simulink model "mpm_blocks"  (R2023a)
settings: Solver=VariableStepAuto  StartTime=0.0  StopTime=10.0  RelTol=1e-3
undefined symbols (not defined in the file or in its folder): conv, es
(part 2 of 3)

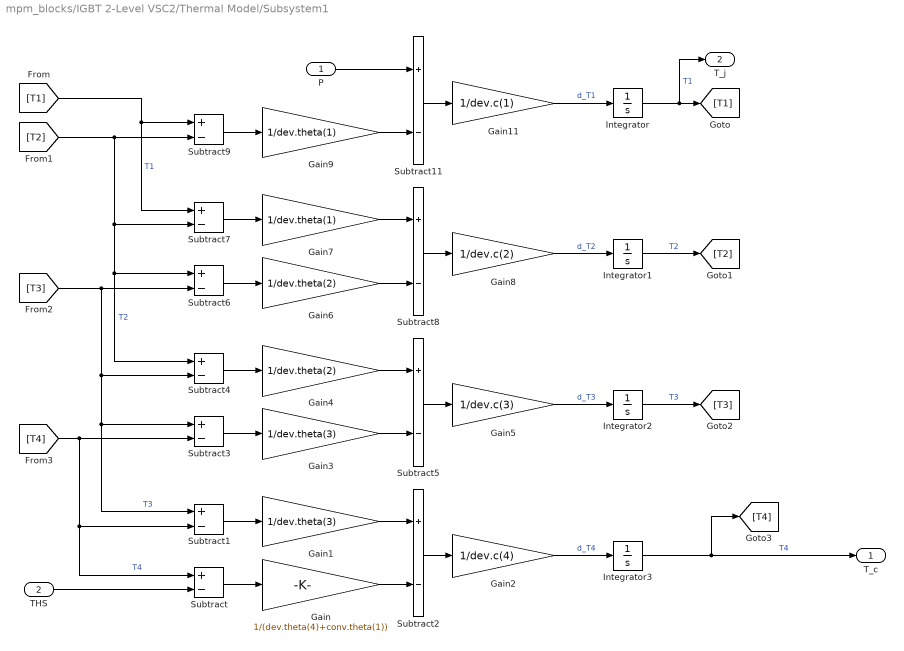
== system mpm_blocks/IGBT 2-Level VSC2/Thermal Model/Subsystem1 ==
  P : Inport
  THS : Inport  Port=2
  Gain : Gain  Gain=1/(dev.theta(4)+conv.theta(1))
  Gain1 : Gain  Gain=1/dev.theta(3)
  Gain11 : Gain  Gain=1/dev.c(1)
  Gain2 : Gain  Gain=1/dev.c(4)
  Gain3 : Gain  Gain=1/dev.theta(3)
  Gain4 : Gain  Gain=1/dev.theta(2)
  Gain5 : Gain  Gain=1/dev.c(3)
  Gain6 : Gain  Gain=1/dev.theta(2)
  Gain7 : Gain  Gain=1/dev.theta(1)
  Gain8 : Gain  Gain=1/dev.c(2)
  Gain9 : Gain  Gain=1/dev.theta(1)
  Integrator{,1..3} (4 alike) : Integrator  InitialCondition=conv.T_init-273.15
  Subtract{,1..9,11} (11 alike) : Sum  Inputs=+-
  T_c : Outport
  T_j : Outport  Port=2
  wires:
  Gain6/1 -> Subtract8/2
  Gain7/1 -> Subtract8/1
  Subtract11/1 -> Gain11/1
  Subtract6/1 -> Gain6/1
  Subtract2/1 -> Gain2/1
  Gain11/1 -> Integrator/1  "d_T1"
  Gain5/1 -> Integrator2/1  "d_T3"
  Integrator2/1 -> [T3]  "T3"
  Gain3/1 -> Subtract5/2
  Gain9/1 -> Subtract11/2
  Gain1/1 -> Subtract2/1
  THS/1 -> Subtract/2
  Subtract8/1 -> Gain8/1
  Gain2/1 -> Integrator3/1  "d_T4"
  Integrator3/1 -> T_c/1, [T4]  "T4"
  Subtract4/1 -> Gain4/1
  Subtract7/1 -> Gain7/1
  [T4] -> Subtract3/2, Subtract1/2, Subtract/1  "T4"
  Subtract/1 -> Gain/1
  Integrator1/1 -> [T2]  "T2"
  [T1] -> Subtract7/1, Subtract9/1  "T1"
  Subtract1/1 -> Gain1/1
  Subtract9/1 -> Gain9/1
  P/1 -> Subtract11/1
  [T3] -> Subtract6/2, Subtract4/2, Subtract3/1, Subtract1/1  "T3"
  Integrator/1 -> [T1], T_j/1  "T1"
  Gain8/1 -> Integrator1/1  "d_T2"
  Subtract3/1 -> Gain3/1
  Gain4/1 -> Subtract5/1
  Subtract5/1 -> Gain5/1
  Gain/1 -> Subtract2/2
  [T2] -> Subtract9/2, Subtract7/2, Subtract6/1, Subtract4/1  "T2"

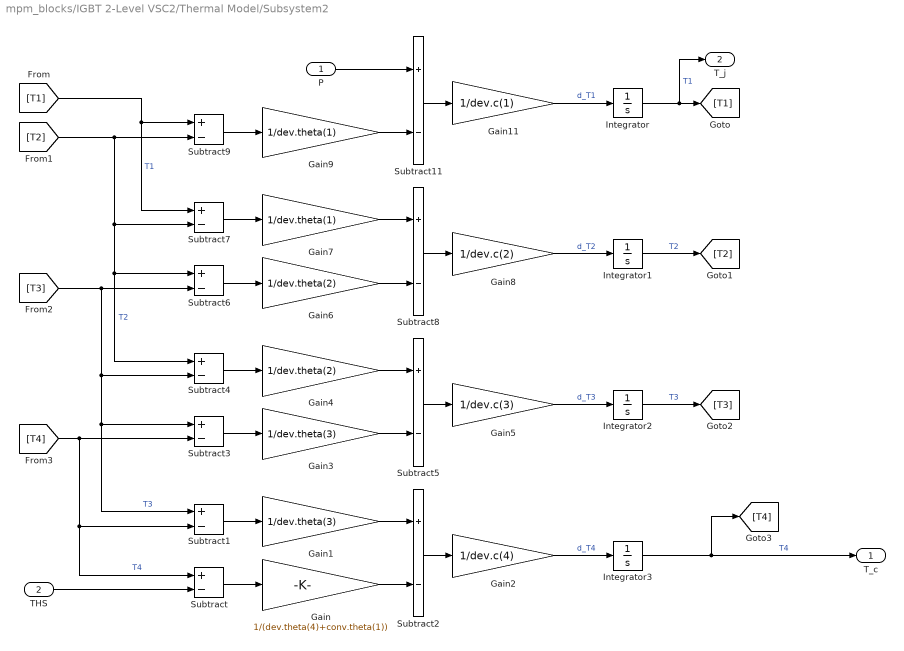
== system mpm_blocks/IGBT 2-Level VSC2/Thermal Model/Subsystem2 ==
  P : Inport
  THS : Inport  Port=2
  Gain : Gain  Gain=1/(dev.theta(4)+conv.theta(1))
  Gain1 : Gain  Gain=1/dev.theta(3)
  Gain11 : Gain  Gain=1/dev.c(1)
  Gain2 : Gain  Gain=1/dev.c(4)
  Gain3 : Gain  Gain=1/dev.theta(3)
  Gain4 : Gain  Gain=1/dev.theta(2)
  Gain5 : Gain  Gain=1/dev.c(3)
  Gain6 : Gain  Gain=1/dev.theta(2)
  Gain7 : Gain  Gain=1/dev.theta(1)
  Gain8 : Gain  Gain=1/dev.c(2)
  Gain9 : Gain  Gain=1/dev.theta(1)
  Integrator{,1..3} (4 alike) : Integrator  InitialCondition=conv.T_init-273.15
  Subtract{,1..9,11} (11 alike) : Sum  Inputs=+-
  T_c : Outport
  T_j : Outport  Port=2
  wires:
  Gain6/1 -> Subtract8/2
  Gain7/1 -> Subtract8/1
  Subtract11/1 -> Gain11/1
  Subtract6/1 -> Gain6/1
  Subtract2/1 -> Gain2/1
  Gain11/1 -> Integrator/1  "d_T1"
  Gain5/1 -> Integrator2/1  "d_T3"
  Integrator2/1 -> [T3]  "T3"
  Gain3/1 -> Subtract5/2
  Gain9/1 -> Subtract11/2
  Gain1/1 -> Subtract2/1
  THS/1 -> Subtract/2
  Subtract8/1 -> Gain8/1
  Gain2/1 -> Integrator3/1  "d_T4"
  Integrator3/1 -> T_c/1, [T4]  "T4"
  Subtract4/1 -> Gain4/1
  Subtract7/1 -> Gain7/1
  [T4] -> Subtract3/2, Subtract1/2, Subtract/1  "T4"
  Subtract/1 -> Gain/1
  Integrator1/1 -> [T2]  "T2"
  [T1] -> Subtract7/1, Subtract9/1  "T1"
  Subtract1/1 -> Gain1/1
  Subtract9/1 -> Gain9/1
  P/1 -> Subtract11/1
  [T3] -> Subtract6/2, Subtract4/2, Subtract3/1, Subtract1/1  "T3"
  Integrator/1 -> [T1], T_j/1  "T1"
  Gain8/1 -> Integrator1/1  "d_T2"
  Subtract3/1 -> Gain3/1
  Gain4/1 -> Subtract5/1
  Subtract5/1 -> Gain5/1
  Gain/1 -> Subtract2/2
  [T2] -> Subtract9/2, Subtract7/2, Subtract6/1, Subtract4/1  "T2"

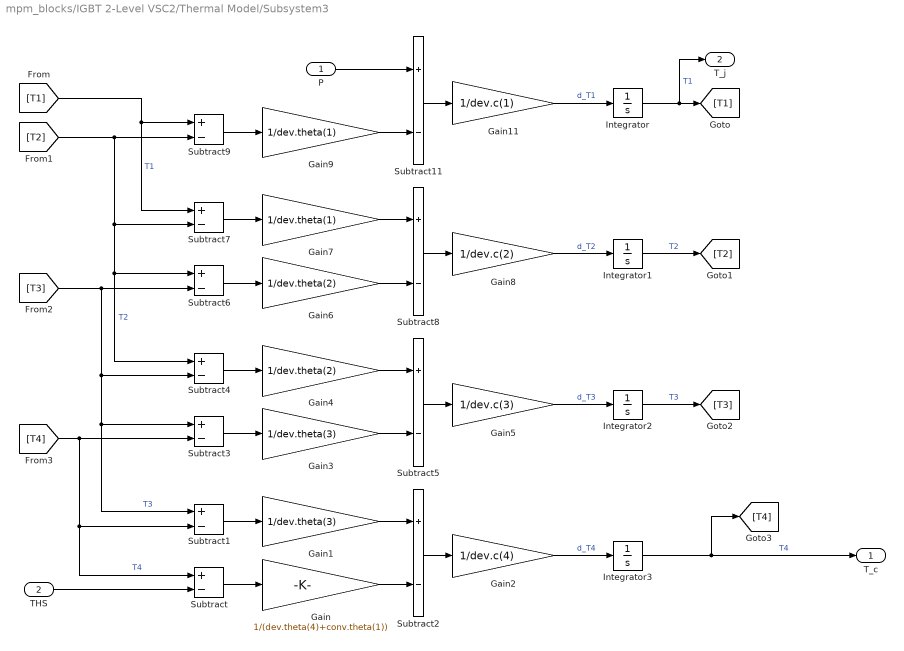
== system mpm_blocks/IGBT 2-Level VSC2/Thermal Model/Subsystem3 ==
  P : Inport
  THS : Inport  Port=2
  Gain : Gain  Gain=1/(dev.theta(4)+conv.theta(1))
  Gain1 : Gain  Gain=1/dev.theta(3)
  Gain11 : Gain  Gain=1/dev.c(1)
  Gain2 : Gain  Gain=1/dev.c(4)
  Gain3 : Gain  Gain=1/dev.theta(3)
  Gain4 : Gain  Gain=1/dev.theta(2)
  Gain5 : Gain  Gain=1/dev.c(3)
  Gain6 : Gain  Gain=1/dev.theta(2)
  Gain7 : Gain  Gain=1/dev.theta(1)
  Gain8 : Gain  Gain=1/dev.c(2)
  Gain9 : Gain  Gain=1/dev.theta(1)
  Integrator{,1..3} (4 alike) : Integrator  InitialCondition=conv.T_init-273.15
  Subtract{,1..9,11} (11 alike) : Sum  Inputs=+-
  T_c : Outport
  T_j : Outport  Port=2
  wires:
  Gain6/1 -> Subtract8/2
  Gain7/1 -> Subtract8/1
  Subtract11/1 -> Gain11/1
  Subtract6/1 -> Gain6/1
  Subtract2/1 -> Gain2/1
  Gain11/1 -> Integrator/1  "d_T1"
  Gain5/1 -> Integrator2/1  "d_T3"
  Integrator2/1 -> [T3]  "T3"
  Gain3/1 -> Subtract5/2
  Gain9/1 -> Subtract11/2
  Gain1/1 -> Subtract2/1
  THS/1 -> Subtract/2
  Subtract8/1 -> Gain8/1
  Gain2/1 -> Integrator3/1  "d_T4"
  Integrator3/1 -> T_c/1, [T4]  "T4"
  Subtract4/1 -> Gain4/1
  Subtract7/1 -> Gain7/1
  [T4] -> Subtract3/2, Subtract1/2, Subtract/1  "T4"
  Subtract/1 -> Gain/1
  Integrator1/1 -> [T2]  "T2"
  [T1] -> Subtract7/1, Subtract9/1  "T1"
  Subtract1/1 -> Gain1/1
  Subtract9/1 -> Gain9/1
  P/1 -> Subtract11/1
  [T3] -> Subtract6/2, Subtract4/2, Subtract3/1, Subtract1/1  "T3"
  Integrator/1 -> [T1], T_j/1  "T1"
  Gain8/1 -> Integrator1/1  "d_T2"
  Subtract3/1 -> Gain3/1
  Gain4/1 -> Subtract5/1
  Subtract5/1 -> Gain5/1
  Gain/1 -> Subtract2/2
  [T2] -> Subtract9/2, Subtract7/2, Subtract6/1, Subtract4/1  "T2"

== system mpm_blocks/IGBT 2-Level VSC2/Thermal Model/Subsystem4 ==
  P : Inport
  THS : Inport  Port=2
  Gain : Gain  Gain=1/(dev.theta(4)+conv.theta(1))
  Gain1 : Gain  Gain=1/dev.theta(3)
  Gain11 : Gain  Gain=1/dev.c(1)
  Gain2 : Gain  Gain=1/dev.c(4)
  Gain3 : Gain  Gain=1/dev.theta(3)
  Gain4 : Gain  Gain=1/dev.theta(2)
  Gain5 : Gain  Gain=1/dev.c(3)
  Gain6 : Gain  Gain=1/dev.theta(2)
  Gain7 : Gain  Gain=1/dev.theta(1)
  Gain8 : Gain  Gain=1/dev.c(2)
  Gain9 : Gain  Gain=1/dev.theta(1)
  Integrator{,1..3} (4 alike) : Integrator  InitialCondition=conv.T_init-273.15
  Subtract{,1..9,11} (11 alike) : Sum  Inputs=+-
  T_c : Outport
  T_j : Outport  Port=2
  wires:
  Gain6/1 -> Subtract8/2
  Gain7/1 -> Subtract8/1
  Subtract11/1 -> Gain11/1
  Subtract6/1 -> Gain6/1
  Subtract2/1 -> Gain2/1
  Gain11/1 -> Integrator/1  "d_T1"
  Gain5/1 -> Integrator2/1  "d_T3"
  Integrator2/1 -> [T3]  "T3"
  Gain3/1 -> Subtract5/2
  Gain9/1 -> Subtract11/2
  Gain1/1 -> Subtract2/1
  THS/1 -> Subtract/2
  Subtract8/1 -> Gain8/1
  Gain2/1 -> Integrator3/1  "d_T4"
  Integrator3/1 -> T_c/1, [T4]  "T4"
  Subtract4/1 -> Gain4/1
  Subtract7/1 -> Gain7/1
  [T4] -> Subtract3/2, Subtract1/2, Subtract/1  "T4"
  Subtract/1 -> Gain/1
  Integrator1/1 -> [T2]  "T2"
  [T1] -> Subtract7/1, Subtract9/1  "T1"
  Subtract1/1 -> Gain1/1
  Subtract9/1 -> Gain9/1
  P/1 -> Subtract11/1
  [T3] -> Subtract6/2, Subtract4/2, Subtract3/1, Subtract1/1  "T3"
  Integrator/1 -> [T1], T_j/1  "T1"
  Gain8/1 -> Integrator1/1  "d_T2"
  Subtract3/1 -> Gain3/1
  Gain4/1 -> Subtract5/1
  Subtract5/1 -> Gain5/1
  Gain/1 -> Subtract2/2
  [T2] -> Subtract9/2, Subtract7/2, Subtract6/1, Subtract4/1  "T2"

== system mpm_blocks/IGBT 2-Level VSC2/Thermal Model/Subsystem5 ==
  P : Inport
  THS : Inport  Port=2
  Gain : Gain  Gain=1/(dev.theta(4)+conv.theta(1))
  Gain1 : Gain  Gain=1/dev.theta(3)
  Gain11 : Gain  Gain=1/dev.c(1)
  Gain2 : Gain  Gain=1/dev.c(4)
  Gain3 : Gain  Gain=1/dev.theta(3)
  Gain4 : Gain  Gain=1/dev.theta(2)
  Gain5 : Gain  Gain=1/dev.c(3)
  Gain6 : Gain  Gain=1/dev.theta(2)
  Gain7 : Gain  Gain=1/dev.theta(1)
  Gain8 : Gain  Gain=1/dev.c(2)
  Gain9 : Gain  Gain=1/dev.theta(1)
  Integrator{,1..3} (4 alike) : Integrator  InitialCondition=conv.T_init-273.15
  Subtract{,1..9,11} (11 alike) : Sum  Inputs=+-
  T_c : Outport
  T_j : Outport  Port=2
  wires:
  Gain6/1 -> Subtract8/2
  Gain7/1 -> Subtract8/1
  Subtract11/1 -> Gain11/1
  Subtract6/1 -> Gain6/1
  Subtract2/1 -> Gain2/1
  Gain11/1 -> Integrator/1  "d_T1"
  Gain5/1 -> Integrator2/1  "d_T3"
  Integrator2/1 -> [T3]  "T3"
  Gain3/1 -> Subtract5/2
  Gain9/1 -> Subtract11/2
  Gain1/1 -> Subtract2/1
  THS/1 -> Subtract/2
  Subtract8/1 -> Gain8/1
  Gain2/1 -> Integrator3/1  "d_T4"
  Integrator3/1 -> T_c/1, [T4]  "T4"
  Subtract4/1 -> Gain4/1
  Subtract7/1 -> Gain7/1
  [T4] -> Subtract3/2, Subtract1/2, Subtract/1  "T4"
  Subtract/1 -> Gain/1
  Integrator1/1 -> [T2]  "T2"
  [T1] -> Subtract7/1, Subtract9/1  "T1"
  Subtract1/1 -> Gain1/1
  Subtract9/1 -> Gain9/1
  P/1 -> Subtract11/1
  [T3] -> Subtract6/2, Subtract4/2, Subtract3/1, Subtract1/1  "T3"
  Integrator/1 -> [T1], T_j/1  "T1"
  Gain8/1 -> Integrator1/1  "d_T2"
  Subtract3/1 -> Gain3/1
  Gain4/1 -> Subtract5/1
  Subtract5/1 -> Gain5/1
  Gain/1 -> Subtract2/2
  [T2] -> Subtract9/2, Subtract7/2, Subtract6/1, Subtract4/1  "T2"

== system mpm_blocks/IGBT 2-Level VSC2/Thermal Model/Subsystem6 ==
  P : Inport
  THS : Inport  Port=2
  Gain : Gain  Gain=1/(dev.theta(4)+conv.theta(1))
  Gain1 : Gain  Gain=1/dev.theta(3)
  Gain11 : Gain  Gain=1/dev.c(1)
  Gain2 : Gain  Gain=1/dev.c(4)
  Gain3 : Gain  Gain=1/dev.theta(3)
  Gain4 : Gain  Gain=1/dev.theta(2)
  Gain5 : Gain  Gain=1/dev.c(3)
  Gain6 : Gain  Gain=1/dev.theta(2)
  Gain7 : Gain  Gain=1/dev.theta(1)
  Gain8 : Gain  Gain=1/dev.c(2)
  Gain9 : Gain  Gain=1/dev.theta(1)
  Integrator{,1..3} (4 alike) : Integrator  InitialCondition=conv.T_init-273.15
  Subtract{,1..9,11} (11 alike) : Sum  Inputs=+-
  T_c : Outport
  T_j : Outport  Port=2
  wires:
  Gain6/1 -> Subtract8/2
  Gain7/1 -> Subtract8/1
  Subtract11/1 -> Gain11/1
  Subtract6/1 -> Gain6/1
  Subtract2/1 -> Gain2/1
  Gain11/1 -> Integrator/1  "d_T1"
  Gain5/1 -> Integrator2/1  "d_T3"
  Integrator2/1 -> [T3]  "T3"
  Gain3/1 -> Subtract5/2
  Gain9/1 -> Subtract11/2
  Gain1/1 -> Subtract2/1
  THS/1 -> Subtract/2
  Subtract8/1 -> Gain8/1
  Gain2/1 -> Integrator3/1  "d_T4"
  Integrator3/1 -> T_c/1, [T4]  "T4"
  Subtract4/1 -> Gain4/1
  Subtract7/1 -> Gain7/1
  [T4] -> Subtract3/2, Subtract1/2, Subtract/1  "T4"
  Subtract/1 -> Gain/1
  Integrator1/1 -> [T2]  "T2"
  [T1] -> Subtract7/1, Subtract9/1  "T1"
  Subtract1/1 -> Gain1/1
  Subtract9/1 -> Gain9/1
  P/1 -> Subtract11/1
  [T3] -> Subtract6/2, Subtract4/2, Subtract3/1, Subtract1/1  "T3"
  Integrator/1 -> [T1], T_j/1  "T1"
  Gain8/1 -> Integrator1/1  "d_T2"
  Subtract3/1 -> Gain3/1
  Gain4/1 -> Subtract5/1
  Subtract5/1 -> Gain5/1
  Gain/1 -> Subtract2/2
  [T2] -> Subtract9/2, Subtract7/2, Subtract6/1, Subtract4/1  "T2"

== system mpm_blocks/IGBT 2-Level VSC2/Thermal Model1/Subsystem1 ==
  P : Inport
  THS : Inport  Port=2
  Gain : Gain  Gain=1/(dev.theta(4)+conv.theta(1))
  Gain1 : Gain  Gain=1/dev.theta(3)
  Gain11 : Gain  Gain=1/dev.c(1)
  Gain2 : Gain  Gain=1/dev.c(4)
  Gain3 : Gain  Gain=1/dev.theta(3)
  Gain4 : Gain  Gain=1/dev.theta(2)
  Gain5 : Gain  Gain=1/dev.c(3)
  Gain6 : Gain  Gain=1/dev.theta(2)
  Gain7 : Gain  Gain=1/dev.theta(1)
  Gain8 : Gain  Gain=1/dev.c(2)
  Gain9 : Gain  Gain=1/dev.theta(1)
  Integrator{,1..3} (4 alike) : Integrator  InitialCondition=conv.T_init-273.15
  Subtract{,1..9,11} (11 alike) : Sum  Inputs=+-
  T_c : Outport
  T_j : Outport  Port=2
  wires:
  [T2] -> Subtract4/1, Subtract6/1, Subtract7/2, Subtract9/2  "T2"
  Gain/1 -> Subtract2/2
  Subtract5/1 -> Gain5/1
  Gain4/1 -> Subtract5/1
  Subtract3/1 -> Gain3/1
  Gain8/1 -> Integrator1/1  "d_T2"
  Integrator/1 -> T_j/1, [T1]  "T1"
  [T3] -> Subtract1/1, Subtract3/1, Subtract4/2, Subtract6/2  "T3"
  P/1 -> Subtract11/1
  Subtract9/1 -> Gain9/1
  Subtract1/1 -> Gain1/1
  [T1] -> Subtract9/1, Subtract7/1  "T1"
  Integrator1/1 -> [T2]  "T2"
  Subtract/1 -> Gain/1
  [T4] -> Subtract/1, Subtract1/2, Subtract3/2  "T4"
  Subtract7/1 -> Gain7/1
  Subtract4/1 -> Gain4/1
  Integrator3/1 -> [T4], T_c/1  "T4"
  Gain2/1 -> Integrator3/1  "d_T4"
  Subtract8/1 -> Gain8/1
  THS/1 -> Subtract/2
  Gain1/1 -> Subtract2/1
  Gain9/1 -> Subtract11/2
  Gain3/1 -> Subtract5/2
  Integrator2/1 -> [T3]  "T3"
  Gain5/1 -> Integrator2/1  "d_T3"
  Gain11/1 -> Integrator/1  "d_T1"
  Subtract2/1 -> Gain2/1
  Subtract6/1 -> Gain6/1
  Subtract11/1 -> Gain11/1
  Gain7/1 -> Subtract8/1
  Gain6/1 -> Subtract8/2

== system mpm_blocks/IGBT 2-Level VSC2/Thermal Model1/Subsystem2 ==
  P : Inport
  THS : Inport  Port=2
  Gain : Gain  Gain=1/(dev.theta(4)+conv.theta(1))
  Gain1 : Gain  Gain=1/dev.theta(3)
  Gain11 : Gain  Gain=1/dev.c(1)
  Gain2 : Gain  Gain=1/dev.c(4)
  Gain3 : Gain  Gain=1/dev.theta(3)
  Gain4 : Gain  Gain=1/dev.theta(2)
  Gain5 : Gain  Gain=1/dev.c(3)
  Gain6 : Gain  Gain=1/dev.theta(2)
  Gain7 : Gain  Gain=1/dev.theta(1)
  Gain8 : Gain  Gain=1/dev.c(2)
  Gain9 : Gain  Gain=1/dev.theta(1)
  Integrator{,1..3} (4 alike) : Integrator  InitialCondition=conv.T_init-273.15
  Subtract{,1..9,11} (11 alike) : Sum  Inputs=+-
  T_c : Outport
  T_j : Outport  Port=2
  wires:
  [T2] -> Subtract4/1, Subtract6/1, Subtract7/2, Subtract9/2  "T2"
  Gain/1 -> Subtract2/2
  Subtract5/1 -> Gain5/1
  Gain4/1 -> Subtract5/1
  Subtract3/1 -> Gain3/1
  Gain8/1 -> Integrator1/1  "d_T2"
  Integrator/1 -> T_j/1, [T1]  "T1"
  [T3] -> Subtract1/1, Subtract3/1, Subtract4/2, Subtract6/2  "T3"
  P/1 -> Subtract11/1
  Subtract9/1 -> Gain9/1
  Subtract1/1 -> Gain1/1
  [T1] -> Subtract9/1, Subtract7/1  "T1"
  Integrator1/1 -> [T2]  "T2"
  Subtract/1 -> Gain/1
  [T4] -> Subtract/1, Subtract1/2, Subtract3/2  "T4"
  Subtract7/1 -> Gain7/1
  Subtract4/1 -> Gain4/1
  Integrator3/1 -> [T4], T_c/1  "T4"
  Gain2/1 -> Integrator3/1  "d_T4"
  Subtract8/1 -> Gain8/1
  THS/1 -> Subtract/2
  Gain1/1 -> Subtract2/1
  Gain9/1 -> Subtract11/2
  Gain3/1 -> Subtract5/2
  Integrator2/1 -> [T3]  "T3"
  Gain5/1 -> Integrator2/1  "d_T3"
  Gain11/1 -> Integrator/1  "d_T1"
  Subtract2/1 -> Gain2/1
  Subtract6/1 -> Gain6/1
  Subtract11/1 -> Gain11/1
  Gain7/1 -> Subtract8/1
  Gain6/1 -> Subtract8/2

== system mpm_blocks/IGBT 2-Level VSC2/Thermal Model1/Subsystem3 ==
  P : Inport
  THS : Inport  Port=2
  Gain : Gain  Gain=1/(dev.theta(4)+conv.theta(1))
  Gain1 : Gain  Gain=1/dev.theta(3)
  Gain11 : Gain  Gain=1/dev.c(1)
  Gain2 : Gain  Gain=1/dev.c(4)
  Gain3 : Gain  Gain=1/dev.theta(3)
  Gain4 : Gain  Gain=1/dev.theta(2)
  Gain5 : Gain  Gain=1/dev.c(3)
  Gain6 : Gain  Gain=1/dev.theta(2)
  Gain7 : Gain  Gain=1/dev.theta(1)
  Gain8 : Gain  Gain=1/dev.c(2)
  Gain9 : Gain  Gain=1/dev.theta(1)
  Integrator{,1..3} (4 alike) : Integrator  InitialCondition=conv.T_init-273.15
  Subtract{,1..9,11} (11 alike) : Sum  Inputs=+-
  T_c : Outport
  T_j : Outport  Port=2
  wires:
  [T2] -> Subtract4/1, Subtract6/1, Subtract7/2, Subtract9/2  "T2"
  Gain/1 -> Subtract2/2
  Subtract5/1 -> Gain5/1
  Gain4/1 -> Subtract5/1
  Subtract3/1 -> Gain3/1
  Gain8/1 -> Integrator1/1  "d_T2"
  Integrator/1 -> T_j/1, [T1]  "T1"
  [T3] -> Subtract1/1, Subtract3/1, Subtract4/2, Subtract6/2  "T3"
  P/1 -> Subtract11/1
  Subtract9/1 -> Gain9/1
  Subtract1/1 -> Gain1/1
  [T1] -> Subtract9/1, Subtract7/1  "T1"
  Integrator1/1 -> [T2]  "T2"
  Subtract/1 -> Gain/1
  [T4] -> Subtract/1, Subtract1/2, Subtract3/2  "T4"
  Subtract7/1 -> Gain7/1
  Subtract4/1 -> Gain4/1
  Integrator3/1 -> [T4], T_c/1  "T4"
  Gain2/1 -> Integrator3/1  "d_T4"
  Subtract8/1 -> Gain8/1
  THS/1 -> Subtract/2
  Gain1/1 -> Subtract2/1
  Gain9/1 -> Subtract11/2
  Gain3/1 -> Subtract5/2
  Integrator2/1 -> [T3]  "T3"
  Gain5/1 -> Integrator2/1  "d_T3"
  Gain11/1 -> Integrator/1  "d_T1"
  Subtract2/1 -> Gain2/1
  Subtract6/1 -> Gain6/1
  Subtract11/1 -> Gain11/1
  Gain7/1 -> Subtract8/1
  Gain6/1 -> Subtract8/2

== system mpm_blocks/IGBT 2-Level VSC2/Thermal Model1/Subsystem4 ==
  P : Inport
  THS : Inport  Port=2
  Gain : Gain  Gain=1/(dev.theta(4)+conv.theta(1))
  Gain1 : Gain  Gain=1/dev.theta(3)
  Gain11 : Gain  Gain=1/dev.c(1)
  Gain2 : Gain  Gain=1/dev.c(4)
  Gain3 : Gain  Gain=1/dev.theta(3)
  Gain4 : Gain  Gain=1/dev.theta(2)
  Gain5 : Gain  Gain=1/dev.c(3)
  Gain6 : Gain  Gain=1/dev.theta(2)
  Gain7 : Gain  Gain=1/dev.theta(1)
  Gain8 : Gain  Gain=1/dev.c(2)
  Gain9 : Gain  Gain=1/dev.theta(1)
  Integrator{,1..3} (4 alike) : Integrator  InitialCondition=conv.T_init-273.15
  Subtract{,1..9,11} (11 alike) : Sum  Inputs=+-
  T_c : Outport
  T_j : Outport  Port=2
  wires:
  [T2] -> Subtract4/1, Subtract6/1, Subtract7/2, Subtract9/2  "T2"
  Gain/1 -> Subtract2/2
  Subtract5/1 -> Gain5/1
  Gain4/1 -> Subtract5/1
  Subtract3/1 -> Gain3/1
  Gain8/1 -> Integrator1/1  "d_T2"
  Integrator/1 -> T_j/1, [T1]  "T1"
  [T3] -> Subtract1/1, Subtract3/1, Subtract4/2, Subtract6/2  "T3"
  P/1 -> Subtract11/1
  Subtract9/1 -> Gain9/1
  Subtract1/1 -> Gain1/1
  [T1] -> Subtract9/1, Subtract7/1  "T1"
  Integrator1/1 -> [T2]  "T2"
  Subtract/1 -> Gain/1
  [T4] -> Subtract/1, Subtract1/2, Subtract3/2  "T4"
  Subtract7/1 -> Gain7/1
  Subtract4/1 -> Gain4/1
  Integrator3/1 -> [T4], T_c/1  "T4"
  Gain2/1 -> Integrator3/1  "d_T4"
  Subtract8/1 -> Gain8/1
  THS/1 -> Subtract/2
  Gain1/1 -> Subtract2/1
  Gain9/1 -> Subtract11/2
  Gain3/1 -> Subtract5/2
  Integrator2/1 -> [T3]  "T3"
  Gain5/1 -> Integrator2/1  "d_T3"
  Gain11/1 -> Integrator/1  "d_T1"
  Subtract2/1 -> Gain2/1
  Subtract6/1 -> Gain6/1
  Subtract11/1 -> Gain11/1
  Gain7/1 -> Subtract8/1
  Gain6/1 -> Subtract8/2

== system mpm_blocks/IGBT 2-Level VSC2/Thermal Model1/Subsystem5 ==
  P : Inport
  THS : Inport  Port=2
  Gain : Gain  Gain=1/(dev.theta(4)+conv.theta(1))
  Gain1 : Gain  Gain=1/dev.theta(3)
  Gain11 : Gain  Gain=1/dev.c(1)
  Gain2 : Gain  Gain=1/dev.c(4)
  Gain3 : Gain  Gain=1/dev.theta(3)
  Gain4 : Gain  Gain=1/dev.theta(2)
  Gain5 : Gain  Gain=1/dev.c(3)
  Gain6 : Gain  Gain=1/dev.theta(2)
  Gain7 : Gain  Gain=1/dev.theta(1)
  Gain8 : Gain  Gain=1/dev.c(2)
  Gain9 : Gain  Gain=1/dev.theta(1)
  Integrator{,1..3} (4 alike) : Integrator  InitialCondition=conv.T_init-273.15
  Subtract{,1..9,11} (11 alike) : Sum  Inputs=+-
  T_c : Outport
  T_j : Outport  Port=2
  wires:
  [T2] -> Subtract4/1, Subtract6/1, Subtract7/2, Subtract9/2  "T2"
  Gain/1 -> Subtract2/2
  Subtract5/1 -> Gain5/1
  Gain4/1 -> Subtract5/1
  Subtract3/1 -> Gain3/1
  Gain8/1 -> Integrator1/1  "d_T2"
  Integrator/1 -> T_j/1, [T1]  "T1"
  [T3] -> Subtract1/1, Subtract3/1, Subtract4/2, Subtract6/2  "T3"
  P/1 -> Subtract11/1
  Subtract9/1 -> Gain9/1
  Subtract1/1 -> Gain1/1
  [T1] -> Subtract9/1, Subtract7/1  "T1"
  Integrator1/1 -> [T2]  "T2"
  Subtract/1 -> Gain/1
  [T4] -> Subtract/1, Subtract1/2, Subtract3/2  "T4"
  Subtract7/1 -> Gain7/1
  Subtract4/1 -> Gain4/1
  Integrator3/1 -> [T4], T_c/1  "T4"
  Gain2/1 -> Integrator3/1  "d_T4"
  Subtract8/1 -> Gain8/1
  THS/1 -> Subtract/2
  Gain1/1 -> Subtract2/1
  Gain9/1 -> Subtract11/2
  Gain3/1 -> Subtract5/2
  Integrator2/1 -> [T3]  "T3"
  Gain5/1 -> Integrator2/1  "d_T3"
  Gain11/1 -> Integrator/1  "d_T1"
  Subtract2/1 -> Gain2/1
  Subtract6/1 -> Gain6/1
  Subtract11/1 -> Gain11/1
  Gain7/1 -> Subtract8/1
  Gain6/1 -> Subtract8/2

== system mpm_blocks/IGBT 2-Level VSC2/Thermal Model1/Subsystem6 ==
  P : Inport
  THS : Inport  Port=2
  Gain : Gain  Gain=1/(dev.theta(4)+conv.theta(1))
  Gain1 : Gain  Gain=1/dev.theta(3)
  Gain11 : Gain  Gain=1/dev.c(1)
  Gain2 : Gain  Gain=1/dev.c(4)
  Gain3 : Gain  Gain=1/dev.theta(3)
  Gain4 : Gain  Gain=1/dev.theta(2)
  Gain5 : Gain  Gain=1/dev.c(3)
  Gain6 : Gain  Gain=1/dev.theta(2)
  Gain7 : Gain  Gain=1/dev.theta(1)
  Gain8 : Gain  Gain=1/dev.c(2)
  Gain9 : Gain  Gain=1/dev.theta(1)
  Integrator{,1..3} (4 alike) : Integrator  InitialCondition=conv.T_init-273.15
  Subtract{,1..9,11} (11 alike) : Sum  Inputs=+-
  T_c : Outport
  T_j : Outport  Port=2
  wires:
  [T2] -> Subtract4/1, Subtract6/1, Subtract7/2, Subtract9/2  "T2"
  Gain/1 -> Subtract2/2
  Subtract5/1 -> Gain5/1
  Gain4/1 -> Subtract5/1
  Subtract3/1 -> Gain3/1
  Gain8/1 -> Integrator1/1  "d_T2"
  Integrator/1 -> T_j/1, [T1]  "T1"
  [T3] -> Subtract1/1, Subtract3/1, Subtract4/2, Subtract6/2  "T3"
  P/1 -> Subtract11/1
  Subtract9/1 -> Gain9/1
  Subtract1/1 -> Gain1/1
  [T1] -> Subtract9/1, Subtract7/1  "T1"
  Integrator1/1 -> [T2]  "T2"
  Subtract/1 -> Gain/1
  [T4] -> Subtract/1, Subtract1/2, Subtract3/2  "T4"
  Subtract7/1 -> Gain7/1
  Subtract4/1 -> Gain4/1
  Integrator3/1 -> [T4], T_c/1  "T4"
  Gain2/1 -> Integrator3/1  "d_T4"
  Subtract8/1 -> Gain8/1
  THS/1 -> Subtract/2
  Gain1/1 -> Subtract2/1
  Gain9/1 -> Subtract11/2
  Gain3/1 -> Subtract5/2
  Integrator2/1 -> [T3]  "T3"
  Gain5/1 -> Integrator2/1  "d_T3"
  Gain11/1 -> Integrator/1  "d_T1"
  Subtract2/1 -> Gain2/1
  Subtract6/1 -> Gain6/1
  Subtract11/1 -> Gain11/1
  Gain7/1 -> Subtract8/1
  Gain6/1 -> Subtract8/2

== system mpm_blocks/MOSFET w// External Diode 2-Level VSC/Calculate Duty & Currents/Duty Cycle Estimation ==
  v_dc : Inport
  v_s : Inport  Port=2
  Constant : Constant
  Constant2 : Constant
  Constant3 : Constant  Value=2*conv.t_d*conv.f_sw
  Constant4 : Constant  Value=2*conv.t_d*conv.f_sw
  Divide : Product  Inputs=*/
  Gain : Gain  Gain=1/2
  Gain2 : Gain  Gain=2
  MATLAB Function : MATLAB Function  Commented=on  TreatAsAtomicUnit=on
  MATLAB Function3 : MATLAB Function  TreatAsAtomicUnit=on
  Mux : Mux  Inputs=[3 3]
  Mux1 : Mux  Inputs=3
  Selector : Selector  InputPortWidth=7  IndexOptions=Index vector (dialog)  Indices=[1 4 7]  OutputSizes=1
  Subtract : Sum  Inputs=-+-
  Sum of Elements : Sum  Inputs=+
  Sum1 : Sum  Inputs=+-+
  d_M : Outport
  d_deadTime : Outport  Port=2
  wires:
  MATLAB Function3/1(y) -> Sum1/3
  Constant/1 -> Sum1/1
  v_s/1 -> Gain2/1  "v_s"
  Constant2/1 -> Subtract/2
  Gain/1 -> Subtract/1, Mux/1, Mux1/1, MATLAB Function/1(d1)  "d_H"
  Divide/1 -> MATLAB Function3/1(u)  "m_a"
  Sum1/1 -> Gain/1
  Constant4/1 -> Mux1/3, MATLAB Function/3(d3), d_deadTime/1, Subtract/3  "d_deadTime"
  Subtract/1 -> Mux/2, Mux1/2, MATLAB Function/2(d2)  "d_L"
  Constant3/1 -> Sum1/2
  Mux/1 -> d_M/1
  Gain2/1 -> Divide/1
  v_dc/1 -> Divide/2
  Mux1/1 -> Selector/1
  Sum of Elements/1 -> ?  "dsum"
  Selector/1 -> Sum of Elements/1

== system mpm_blocks/MOSFET w// External Diode 2-Level VSC/Thermal Model/Subsystem1 ==
  P : Inport
  THS : Inport  Port=2
  Gain : Gain  Gain=1/(dev.theta(4)+conv.theta(1))
  Gain1 : Gain  Gain=1/dev.theta(3)
  Gain11 : Gain  Gain=1/dev.c(1)
  Gain2 : Gain  Gain=1/dev.c(4)
  Gain3 : Gain  Gain=1/dev.theta(3)
  Gain4 : Gain  Gain=1/dev.theta(2)
  Gain5 : Gain  Gain=1/dev.c(3)
  Gain6 : Gain  Gain=1/dev.theta(2)
  Gain7 : Gain  Gain=1/dev.theta(1)
  Gain8 : Gain  Gain=1/dev.c(2)
  Gain9 : Gain  Gain=1/dev.theta(1)
  Integrator{,1..3} (4 alike) : Integrator  InitialCondition=conv.T_init-273.15
  Subtract{,1..9,11} (11 alike) : Sum  Inputs=+-
  T_c : Outport
  T_j : Outport  Port=2
  wires:
  [T2] -> Subtract4/1, Subtract6/1, Subtract7/2, Subtract9/2  "T2"
  Gain/1 -> Subtract2/2
  Subtract5/1 -> Gain5/1
  Gain4/1 -> Subtract5/1
  Subtract3/1 -> Gain3/1
  Gain8/1 -> Integrator1/1  "d_T2"
  Integrator/1 -> T_j/1, [T1]  "T1"
  [T3] -> Subtract1/1, Subtract3/1, Subtract4/2, Subtract6/2  "T3"
  P/1 -> Subtract11/1
  Subtract9/1 -> Gain9/1
  Subtract1/1 -> Gain1/1
  [T1] -> Subtract9/1, Subtract7/1  "T1"
  Integrator1/1 -> [T2]  "T2"
  Subtract/1 -> Gain/1
  [T4] -> Subtract/1, Subtract1/2, Subtract3/2  "T4"
  Subtract7/1 -> Gain7/1
  Subtract4/1 -> Gain4/1
  Integrator3/1 -> [T4], T_c/1  "T4"
  Gain2/1 -> Integrator3/1  "d_T4"
  Subtract8/1 -> Gain8/1
  THS/1 -> Subtract/2
  Gain1/1 -> Subtract2/1
  Gain9/1 -> Subtract11/2
  Gain3/1 -> Subtract5/2
  Integrator2/1 -> [T3]  "T3"
  Gain5/1 -> Integrator2/1  "d_T3"
  Gain11/1 -> Integrator/1  "d_T1"
  Subtract2/1 -> Gain2/1
  Subtract6/1 -> Gain6/1
  Subtract11/1 -> Gain11/1
  Gain7/1 -> Subtract8/1
  Gain6/1 -> Subtract8/2

== system mpm_blocks/MOSFET w// External Diode 2-Level VSC/Thermal Model/Subsystem2 ==
  P : Inport
  THS : Inport  Port=2
  Gain : Gain  Gain=1/(dev.theta(4)+conv.theta(1))
  Gain1 : Gain  Gain=1/dev.theta(3)
  Gain11 : Gain  Gain=1/dev.c(1)
  Gain2 : Gain  Gain=1/dev.c(4)
  Gain3 : Gain  Gain=1/dev.theta(3)
  Gain4 : Gain  Gain=1/dev.theta(2)
  Gain5 : Gain  Gain=1/dev.c(3)
  Gain6 : Gain  Gain=1/dev.theta(2)
  Gain7 : Gain  Gain=1/dev.theta(1)
  Gain8 : Gain  Gain=1/dev.c(2)
  Gain9 : Gain  Gain=1/dev.theta(1)
  Integrator{,1..3} (4 alike) : Integrator  InitialCondition=conv.T_init-273.15
  Subtract{,1..9,11} (11 alike) : Sum  Inputs=+-
  T_c : Outport
  T_j : Outport  Port=2
  wires:
  [T2] -> Subtract4/1, Subtract6/1, Subtract7/2, Subtract9/2  "T2"
  Gain/1 -> Subtract2/2
  Subtract5/1 -> Gain5/1
  Gain4/1 -> Subtract5/1
  Subtract3/1 -> Gain3/1
  Gain8/1 -> Integrator1/1  "d_T2"
  Integrator/1 -> T_j/1, [T1]  "T1"
  [T3] -> Subtract1/1, Subtract3/1, Subtract4/2, Subtract6/2  "T3"
  P/1 -> Subtract11/1
  Subtract9/1 -> Gain9/1
  Subtract1/1 -> Gain1/1
  [T1] -> Subtract9/1, Subtract7/1  "T1"
  Integrator1/1 -> [T2]  "T2"
  Subtract/1 -> Gain/1
  [T4] -> Subtract/1, Subtract1/2, Subtract3/2  "T4"
  Subtract7/1 -> Gain7/1
  Subtract4/1 -> Gain4/1
  Integrator3/1 -> [T4], T_c/1  "T4"
  Gain2/1 -> Integrator3/1  "d_T4"
  Subtract8/1 -> Gain8/1
  THS/1 -> Subtract/2
  Gain1/1 -> Subtract2/1
  Gain9/1 -> Subtract11/2
  Gain3/1 -> Subtract5/2
  Integrator2/1 -> [T3]  "T3"
  Gain5/1 -> Integrator2/1  "d_T3"
  Gain11/1 -> Integrator/1  "d_T1"
  Subtract2/1 -> Gain2/1
  Subtract6/1 -> Gain6/1
  Subtract11/1 -> Gain11/1
  Gain7/1 -> Subtract8/1
  Gain6/1 -> Subtract8/2

== system mpm_blocks/MOSFET w// External Diode 2-Level VSC/Thermal Model/Subsystem3 ==
  P : Inport
  THS : Inport  Port=2
  Gain : Gain  Gain=1/(dev.theta(4)+conv.theta(1))
  Gain1 : Gain  Gain=1/dev.theta(3)
  Gain11 : Gain  Gain=1/dev.c(1)
  Gain2 : Gain  Gain=1/dev.c(4)
  Gain3 : Gain  Gain=1/dev.theta(3)
  Gain4 : Gain  Gain=1/dev.theta(2)
  Gain5 : Gain  Gain=1/dev.c(3)
  Gain6 : Gain  Gain=1/dev.theta(2)
  Gain7 : Gain  Gain=1/dev.theta(1)
  Gain8 : Gain  Gain=1/dev.c(2)
  Gain9 : Gain  Gain=1/dev.theta(1)
  Integrator{,1..3} (4 alike) : Integrator  InitialCondition=conv.T_init-273.15
  Subtract{,1..9,11} (11 alike) : Sum  Inputs=+-
  T_c : Outport
  T_j : Outport  Port=2
  wires:
  [T2] -> Subtract4/1, Subtract6/1, Subtract7/2, Subtract9/2  "T2"
  Gain/1 -> Subtract2/2
  Subtract5/1 -> Gain5/1
  Gain4/1 -> Subtract5/1
  Subtract3/1 -> Gain3/1
  Gain8/1 -> Integrator1/1  "d_T2"
  Integrator/1 -> T_j/1, [T1]  "T1"
  [T3] -> Subtract1/1, Subtract3/1, Subtract4/2, Subtract6/2  "T3"
  P/1 -> Subtract11/1
  Subtract9/1 -> Gain9/1
  Subtract1/1 -> Gain1/1
  [T1] -> Subtract9/1, Subtract7/1  "T1"
  Integrator1/1 -> [T2]  "T2"
  Subtract/1 -> Gain/1
  [T4] -> Subtract/1, Subtract1/2, Subtract3/2  "T4"
  Subtract7/1 -> Gain7/1
  Subtract4/1 -> Gain4/1
  Integrator3/1 -> [T4], T_c/1  "T4"
  Gain2/1 -> Integrator3/1  "d_T4"
  Subtract8/1 -> Gain8/1
  THS/1 -> Subtract/2
  Gain1/1 -> Subtract2/1
  Gain9/1 -> Subtract11/2
  Gain3/1 -> Subtract5/2
  Integrator2/1 -> [T3]  "T3"
  Gain5/1 -> Integrator2/1  "d_T3"
  Gain11/1 -> Integrator/1  "d_T1"
  Subtract2/1 -> Gain2/1
  Subtract6/1 -> Gain6/1
  Subtract11/1 -> Gain11/1
  Gain7/1 -> Subtract8/1
  Gain6/1 -> Subtract8/2

== system mpm_blocks/MOSFET w// External Diode 2-Level VSC/Thermal Model/Subsystem4 ==
  P : Inport
  THS : Inport  Port=2
  Gain : Gain  Gain=1/(dev.theta(4)+conv.theta(1))
  Gain1 : Gain  Gain=1/dev.theta(3)
  Gain11 : Gain  Gain=1/dev.c(1)
  Gain2 : Gain  Gain=1/dev.c(4)
  Gain3 : Gain  Gain=1/dev.theta(3)
  Gain4 : Gain  Gain=1/dev.theta(2)
  Gain5 : Gain  Gain=1/dev.c(3)
  Gain6 : Gain  Gain=1/dev.theta(2)
  Gain7 : Gain  Gain=1/dev.theta(1)
  Gain8 : Gain  Gain=1/dev.c(2)
  Gain9 : Gain  Gain=1/dev.theta(1)
  Integrator{,1..3} (4 alike) : Integrator  InitialCondition=conv.T_init-273.15
  Subtract{,1..9,11} (11 alike) : Sum  Inputs=+-
  T_c : Outport
  T_j : Outport  Port=2
  wires:
  [T2] -> Subtract4/1, Subtract6/1, Subtract7/2, Subtract9/2  "T2"
  Gain/1 -> Subtract2/2
  Subtract5/1 -> Gain5/1
  Gain4/1 -> Subtract5/1
  Subtract3/1 -> Gain3/1
  Gain8/1 -> Integrator1/1  "d_T2"
  Integrator/1 -> T_j/1, [T1]  "T1"
  [T3] -> Subtract1/1, Subtract3/1, Subtract4/2, Subtract6/2  "T3"
  P/1 -> Subtract11/1
  Subtract9/1 -> Gain9/1
  Subtract1/1 -> Gain1/1
  [T1] -> Subtract9/1, Subtract7/1  "T1"
  Integrator1/1 -> [T2]  "T2"
  Subtract/1 -> Gain/1
  [T4] -> Subtract/1, Subtract1/2, Subtract3/2  "T4"
  Subtract7/1 -> Gain7/1
  Subtract4/1 -> Gain4/1
  Integrator3/1 -> [T4], T_c/1  "T4"
  Gain2/1 -> Integrator3/1  "d_T4"
  Subtract8/1 -> Gain8/1
  THS/1 -> Subtract/2
  Gain1/1 -> Subtract2/1
  Gain9/1 -> Subtract11/2
  Gain3/1 -> Subtract5/2
  Integrator2/1 -> [T3]  "T3"
  Gain5/1 -> Integrator2/1  "d_T3"
  Gain11/1 -> Integrator/1  "d_T1"
  Subtract2/1 -> Gain2/1
  Subtract6/1 -> Gain6/1
  Subtract11/1 -> Gain11/1
  Gain7/1 -> Subtract8/1
  Gain6/1 -> Subtract8/2

== system mpm_blocks/MOSFET w// External Diode 2-Level VSC/Thermal Model/Subsystem5 ==
  P : Inport
  THS : Inport  Port=2
  Gain : Gain  Gain=1/(dev.theta(4)+conv.theta(1))
  Gain1 : Gain  Gain=1/dev.theta(3)
  Gain11 : Gain  Gain=1/dev.c(1)
  Gain2 : Gain  Gain=1/dev.c(4)
  Gain3 : Gain  Gain=1/dev.theta(3)
  Gain4 : Gain  Gain=1/dev.theta(2)
  Gain5 : Gain  Gain=1/dev.c(3)
  Gain6 : Gain  Gain=1/dev.theta(2)
  Gain7 : Gain  Gain=1/dev.theta(1)
  Gain8 : Gain  Gain=1/dev.c(2)
  Gain9 : Gain  Gain=1/dev.theta(1)
  Integrator{,1..3} (4 alike) : Integrator  InitialCondition=conv.T_init-273.15
  Subtract{,1..9,11} (11 alike) : Sum  Inputs=+-
  T_c : Outport
  T_j : Outport  Port=2
  wires:
  [T2] -> Subtract4/1, Subtract6/1, Subtract7/2, Subtract9/2  "T2"
  Gain/1 -> Subtract2/2
  Subtract5/1 -> Gain5/1
  Gain4/1 -> Subtract5/1
  Subtract3/1 -> Gain3/1
  Gain8/1 -> Integrator1/1  "d_T2"
  Integrator/1 -> T_j/1, [T1]  "T1"
  [T3] -> Subtract1/1, Subtract3/1, Subtract4/2, Subtract6/2  "T3"
  P/1 -> Subtract11/1
  Subtract9/1 -> Gain9/1
  Subtract1/1 -> Gain1/1
  [T1] -> Subtract9/1, Subtract7/1  "T1"
  Integrator1/1 -> [T2]  "T2"
  Subtract/1 -> Gain/1
  [T4] -> Subtract/1, Subtract1/2, Subtract3/2  "T4"
  Subtract7/1 -> Gain7/1
  Subtract4/1 -> Gain4/1
  Integrator3/1 -> [T4], T_c/1  "T4"
  Gain2/1 -> Integrator3/1  "d_T4"
  Subtract8/1 -> Gain8/1
  THS/1 -> Subtract/2
  Gain1/1 -> Subtract2/1
  Gain9/1 -> Subtract11/2
  Gain3/1 -> Subtract5/2
  Integrator2/1 -> [T3]  "T3"
  Gain5/1 -> Integrator2/1  "d_T3"
  Gain11/1 -> Integrator/1  "d_T1"
  Subtract2/1 -> Gain2/1
  Subtract6/1 -> Gain6/1
  Subtract11/1 -> Gain11/1
  Gain7/1 -> Subtract8/1
  Gain6/1 -> Subtract8/2

== system mpm_blocks/MOSFET w// External Diode 2-Level VSC/Thermal Model/Subsystem6 ==
  P : Inport
  THS : Inport  Port=2
  Gain : Gain  Gain=1/(dev.theta(4)+conv.theta(1))
  Gain1 : Gain  Gain=1/dev.theta(3)
  Gain11 : Gain  Gain=1/dev.c(1)
  Gain2 : Gain  Gain=1/dev.c(4)
  Gain3 : Gain  Gain=1/dev.theta(3)
  Gain4 : Gain  Gain=1/dev.theta(2)
  Gain5 : Gain  Gain=1/dev.c(3)
  Gain6 : Gain  Gain=1/dev.theta(2)
  Gain7 : Gain  Gain=1/dev.theta(1)
  Gain8 : Gain  Gain=1/dev.c(2)
  Gain9 : Gain  Gain=1/dev.theta(1)
  Integrator{,1..3} (4 alike) : Integrator  InitialCondition=conv.T_init-273.15
  Subtract{,1..9,11} (11 alike) : Sum  Inputs=+-
  T_c : Outport
  T_j : Outport  Port=2
  wires:
  [T2] -> Subtract4/1, Subtract6/1, Subtract7/2, Subtract9/2  "T2"
  Gain/1 -> Subtract2/2
  Subtract5/1 -> Gain5/1
  Gain4/1 -> Subtract5/1
  Subtract3/1 -> Gain3/1
  Gain8/1 -> Integrator1/1  "d_T2"
  Integrator/1 -> T_j/1, [T1]  "T1"
  [T3] -> Subtract1/1, Subtract3/1, Subtract4/2, Subtract6/2  "T3"
  P/1 -> Subtract11/1
  Subtract9/1 -> Gain9/1
  Subtract1/1 -> Gain1/1
  [T1] -> Subtract9/1, Subtract7/1  "T1"
  Integrator1/1 -> [T2]  "T2"
  Subtract/1 -> Gain/1
  [T4] -> Subtract/1, Subtract1/2, Subtract3/2  "T4"
  Subtract7/1 -> Gain7/1
  Subtract4/1 -> Gain4/1
  Integrator3/1 -> [T4], T_c/1  "T4"
  Gain2/1 -> Integrator3/1  "d_T4"
  Subtract8/1 -> Gain8/1
  THS/1 -> Subtract/2
  Gain1/1 -> Subtract2/1
  Gain9/1 -> Subtract11/2
  Gain3/1 -> Subtract5/2
  Integrator2/1 -> [T3]  "T3"
  Gain5/1 -> Integrator2/1  "d_T3"
  Gain11/1 -> Integrator/1  "d_T1"
  Subtract2/1 -> Gain2/1
  Subtract6/1 -> Gain6/1
  Subtract11/1 -> Gain11/1
  Gain7/1 -> Subtract8/1
  Gain6/1 -> Subtract8/2

== system mpm_blocks/MOSFET w// External Diode 2-Level VSC/Thermal Model 1/Subsystem1 ==
  P : Inport
  THS : Inport  Port=2
  Gain : Gain  Gain=1/(dev.theta(4)+conv.theta(1))
  Gain1 : Gain  Gain=1/dev.theta(3)
  Gain11 : Gain  Gain=1/dev.c(1)
  Gain2 : Gain  Gain=1/dev.c(4)
  Gain3 : Gain  Gain=1/dev.theta(3)
  Gain4 : Gain  Gain=1/dev.theta(2)
  Gain5 : Gain  Gain=1/dev.c(3)
  Gain6 : Gain  Gain=1/dev.theta(2)
  Gain7 : Gain  Gain=1/dev.theta(1)
  Gain8 : Gain  Gain=1/dev.c(2)
  Gain9 : Gain  Gain=1/dev.theta(1)
  Integrator{,1..3} (4 alike) : Integrator  InitialCondition=conv.T_init-273.15
  Subtract{,1..9,11} (11 alike) : Sum  Inputs=+-
  T_c : Outport
  T_j : Outport  Port=2
  wires:
  [T2] -> Subtract4/1, Subtract6/1, Subtract7/2, Subtract9/2  "T2"
  Gain/1 -> Subtract2/2
  Subtract5/1 -> Gain5/1
  Gain4/1 -> Subtract5/1
  Subtract3/1 -> Gain3/1
  Gain8/1 -> Integrator1/1  "d_T2"
  Integrator/1 -> T_j/1, [T1]  "T1"
  [T3] -> Subtract1/1, Subtract3/1, Subtract4/2, Subtract6/2  "T3"
  P/1 -> Subtract11/1
  Subtract9/1 -> Gain9/1
  Subtract1/1 -> Gain1/1
  [T1] -> Subtract9/1, Subtract7/1  "T1"
  Integrator1/1 -> [T2]  "T2"
  Subtract/1 -> Gain/1
  [T4] -> Subtract/1, Subtract1/2, Subtract3/2  "T4"
  Subtract7/1 -> Gain7/1
  Subtract4/1 -> Gain4/1
  Integrator3/1 -> [T4], T_c/1  "T4"
  Gain2/1 -> Integrator3/1  "d_T4"
  Subtract8/1 -> Gain8/1
  THS/1 -> Subtract/2
  Gain1/1 -> Subtract2/1
  Gain9/1 -> Subtract11/2
  Gain3/1 -> Subtract5/2
  Integrator2/1 -> [T3]  "T3"
  Gain5/1 -> Integrator2/1  "d_T3"
  Gain11/1 -> Integrator/1  "d_T1"
  Subtract2/1 -> Gain2/1
  Subtract6/1 -> Gain6/1
  Subtract11/1 -> Gain11/1
  Gain7/1 -> Subtract8/1
  Gain6/1 -> Subtract8/2

== system mpm_blocks/MOSFET w// External Diode 2-Level VSC/Thermal Model 1/Subsystem2 ==
  P : Inport
  THS : Inport  Port=2
  Gain : Gain  Gain=1/(dev.theta(4)+conv.theta(1))
  Gain1 : Gain  Gain=1/dev.theta(3)
  Gain11 : Gain  Gain=1/dev.c(1)
  Gain2 : Gain  Gain=1/dev.c(4)
  Gain3 : Gain  Gain=1/dev.theta(3)
  Gain4 : Gain  Gain=1/dev.theta(2)
  Gain5 : Gain  Gain=1/dev.c(3)
  Gain6 : Gain  Gain=1/dev.theta(2)
  Gain7 : Gain  Gain=1/dev.theta(1)
  Gain8 : Gain  Gain=1/dev.c(2)
  Gain9 : Gain  Gain=1/dev.theta(1)
  Integrator{,1..3} (4 alike) : Integrator  InitialCondition=conv.T_init-273.15
  Subtract{,1..9,11} (11 alike) : Sum  Inputs=+-
  T_c : Outport
  T_j : Outport  Port=2
  wires:
  [T2] -> Subtract4/1, Subtract6/1, Subtract7/2, Subtract9/2  "T2"
  Gain/1 -> Subtract2/2
  Subtract5/1 -> Gain5/1
  Gain4/1 -> Subtract5/1
  Subtract3/1 -> Gain3/1
  Gain8/1 -> Integrator1/1  "d_T2"
  Integrator/1 -> T_j/1, [T1]  "T1"
  [T3] -> Subtract1/1, Subtract3/1, Subtract4/2, Subtract6/2  "T3"
  P/1 -> Subtract11/1
  Subtract9/1 -> Gain9/1
  Subtract1/1 -> Gain1/1
  [T1] -> Subtract9/1, Subtract7/1  "T1"
  Integrator1/1 -> [T2]  "T2"
  Subtract/1 -> Gain/1
  [T4] -> Subtract/1, Subtract1/2, Subtract3/2  "T4"
  Subtract7/1 -> Gain7/1
  Subtract4/1 -> Gain4/1
  Integrator3/1 -> [T4], T_c/1  "T4"
  Gain2/1 -> Integrator3/1  "d_T4"
  Subtract8/1 -> Gain8/1
  THS/1 -> Subtract/2
  Gain1/1 -> Subtract2/1
  Gain9/1 -> Subtract11/2
  Gain3/1 -> Subtract5/2
  Integrator2/1 -> [T3]  "T3"
  Gain5/1 -> Integrator2/1  "d_T3"
  Gain11/1 -> Integrator/1  "d_T1"
  Subtract2/1 -> Gain2/1
  Subtract6/1 -> Gain6/1
  Subtract11/1 -> Gain11/1
  Gain7/1 -> Subtract8/1
  Gain6/1 -> Subtract8/2

== system mpm_blocks/MOSFET w// External Diode 2-Level VSC/Thermal Model 1/Subsystem3 ==
  P : Inport
  THS : Inport  Port=2
  Gain : Gain  Gain=1/(dev.theta(4)+conv.theta(1))
  Gain1 : Gain  Gain=1/dev.theta(3)
  Gain11 : Gain  Gain=1/dev.c(1)
  Gain2 : Gain  Gain=1/dev.c(4)
  Gain3 : Gain  Gain=1/dev.theta(3)
  Gain4 : Gain  Gain=1/dev.theta(2)
  Gain5 : Gain  Gain=1/dev.c(3)
  Gain6 : Gain  Gain=1/dev.theta(2)
  Gain7 : Gain  Gain=1/dev.theta(1)
  Gain8 : Gain  Gain=1/dev.c(2)
  Gain9 : Gain  Gain=1/dev.theta(1)
  Integrator{,1..3} (4 alike) : Integrator  InitialCondition=conv.T_init-273.15
  Subtract{,1..9,11} (11 alike) : Sum  Inputs=+-
  T_c : Outport
  T_j : Outport  Port=2
  wires:
  [T2] -> Subtract4/1, Subtract6/1, Subtract7/2, Subtract9/2  "T2"
  Gain/1 -> Subtract2/2
  Subtract5/1 -> Gain5/1
  Gain4/1 -> Subtract5/1
  Subtract3/1 -> Gain3/1
  Gain8/1 -> Integrator1/1  "d_T2"
  Integrator/1 -> T_j/1, [T1]  "T1"
  [T3] -> Subtract1/1, Subtract3/1, Subtract4/2, Subtract6/2  "T3"
  P/1 -> Subtract11/1
  Subtract9/1 -> Gain9/1
  Subtract1/1 -> Gain1/1
  [T1] -> Subtract9/1, Subtract7/1  "T1"
  Integrator1/1 -> [T2]  "T2"
  Subtract/1 -> Gain/1
  [T4] -> Subtract/1, Subtract1/2, Subtract3/2  "T4"
  Subtract7/1 -> Gain7/1
  Subtract4/1 -> Gain4/1
  Integrator3/1 -> [T4], T_c/1  "T4"
  Gain2/1 -> Integrator3/1  "d_T4"
  Subtract8/1 -> Gain8/1
  THS/1 -> Subtract/2
  Gain1/1 -> Subtract2/1
  Gain9/1 -> Subtract11/2
  Gain3/1 -> Subtract5/2
  Integrator2/1 -> [T3]  "T3"
  Gain5/1 -> Integrator2/1  "d_T3"
  Gain11/1 -> Integrator/1  "d_T1"
  Subtract2/1 -> Gain2/1
  Subtract6/1 -> Gain6/1
  Subtract11/1 -> Gain11/1
  Gain7/1 -> Subtract8/1
  Gain6/1 -> Subtract8/2

== system mpm_blocks/MOSFET w// External Diode 2-Level VSC/Thermal Model 1/Subsystem4 ==
  P : Inport
  THS : Inport  Port=2
  Gain : Gain  Gain=1/(dev.theta(4)+conv.theta(1))
  Gain1 : Gain  Gain=1/dev.theta(3)
  Gain11 : Gain  Gain=1/dev.c(1)
  Gain2 : Gain  Gain=1/dev.c(4)
  Gain3 : Gain  Gain=1/dev.theta(3)
  Gain4 : Gain  Gain=1/dev.theta(2)
  Gain5 : Gain  Gain=1/dev.c(3)
  Gain6 : Gain  Gain=1/dev.theta(2)
  Gain7 : Gain  Gain=1/dev.theta(1)
  Gain8 : Gain  Gain=1/dev.c(2)
  Gain9 : Gain  Gain=1/dev.theta(1)
  Integrator{,1..3} (4 alike) : Integrator  InitialCondition=conv.T_init-273.15
  Subtract{,1..9,11} (11 alike) : Sum  Inputs=+-
  T_c : Outport
  T_j : Outport  Port=2
  wires:
  [T2] -> Subtract4/1, Subtract6/1, Subtract7/2, Subtract9/2  "T2"
  Gain/1 -> Subtract2/2
  Subtract5/1 -> Gain5/1
  Gain4/1 -> Subtract5/1
  Subtract3/1 -> Gain3/1
  Gain8/1 -> Integrator1/1  "d_T2"
  Integrator/1 -> T_j/1, [T1]  "T1"
  [T3] -> Subtract1/1, Subtract3/1, Subtract4/2, Subtract6/2  "T3"
  P/1 -> Subtract11/1
  Subtract9/1 -> Gain9/1
  Subtract1/1 -> Gain1/1
  [T1] -> Subtract9/1, Subtract7/1  "T1"
  Integrator1/1 -> [T2]  "T2"
  Subtract/1 -> Gain/1
  [T4] -> Subtract/1, Subtract1/2, Subtract3/2  "T4"
  Subtract7/1 -> Gain7/1
  Subtract4/1 -> Gain4/1
  Integrator3/1 -> [T4], T_c/1  "T4"
  Gain2/1 -> Integrator3/1  "d_T4"
  Subtract8/1 -> Gain8/1
  THS/1 -> Subtract/2
  Gain1/1 -> Subtract2/1
  Gain9/1 -> Subtract11/2
  Gain3/1 -> Subtract5/2
  Integrator2/1 -> [T3]  "T3"
  Gain5/1 -> Integrator2/1  "d_T3"
  Gain11/1 -> Integrator/1  "d_T1"
  Subtract2/1 -> Gain2/1
  Subtract6/1 -> Gain6/1
  Subtract11/1 -> Gain11/1
  Gain7/1 -> Subtract8/1
  Gain6/1 -> Subtract8/2

== system mpm_blocks/MOSFET w// External Diode 2-Level VSC/Thermal Model 1/Subsystem5 ==
  P : Inport
  THS : Inport  Port=2
  Gain : Gain  Gain=1/(dev.theta(4)+conv.theta(1))
  Gain1 : Gain  Gain=1/dev.theta(3)
  Gain11 : Gain  Gain=1/dev.c(1)
  Gain2 : Gain  Gain=1/dev.c(4)
  Gain3 : Gain  Gain=1/dev.theta(3)
  Gain4 : Gain  Gain=1/dev.theta(2)
  Gain5 : Gain  Gain=1/dev.c(3)
  Gain6 : Gain  Gain=1/dev.theta(2)
  Gain7 : Gain  Gain=1/dev.theta(1)
  Gain8 : Gain  Gain=1/dev.c(2)
  Gain9 : Gain  Gain=1/dev.theta(1)
  Integrator{,1..3} (4 alike) : Integrator  InitialCondition=conv.T_init-273.15
  Subtract{,1..9,11} (11 alike) : Sum  Inputs=+-
  T_c : Outport
  T_j : Outport  Port=2
  wires:
  [T2] -> Subtract4/1, Subtract6/1, Subtract7/2, Subtract9/2  "T2"
  Gain/1 -> Subtract2/2
  Subtract5/1 -> Gain5/1
  Gain4/1 -> Subtract5/1
  Subtract3/1 -> Gain3/1
  Gain8/1 -> Integrator1/1  "d_T2"
  Integrator/1 -> T_j/1, [T1]  "T1"
  [T3] -> Subtract1/1, Subtract3/1, Subtract4/2, Subtract6/2  "T3"
  P/1 -> Subtract11/1
  Subtract9/1 -> Gain9/1
  Subtract1/1 -> Gain1/1
  [T1] -> Subtract9/1, Subtract7/1  "T1"
  Integrator1/1 -> [T2]  "T2"
  Subtract/1 -> Gain/1
  [T4] -> Subtract/1, Subtract1/2, Subtract3/2  "T4"
  Subtract7/1 -> Gain7/1
  Subtract4/1 -> Gain4/1
  Integrator3/1 -> [T4], T_c/1  "T4"
  Gain2/1 -> Integrator3/1  "d_T4"
  Subtract8/1 -> Gain8/1
  THS/1 -> Subtract/2
  Gain1/1 -> Subtract2/1
  Gain9/1 -> Subtract11/2
  Gain3/1 -> Subtract5/2
  Integrator2/1 -> [T3]  "T3"
  Gain5/1 -> Integrator2/1  "d_T3"
  Gain11/1 -> Integrator/1  "d_T1"
  Subtract2/1 -> Gain2/1
  Subtract6/1 -> Gain6/1
  Subtract11/1 -> Gain11/1
  Gain7/1 -> Subtract8/1
  Gain6/1 -> Subtract8/2

== system mpm_blocks/MOSFET w// External Diode 2-Level VSC/Thermal Model 1/Subsystem6 ==
  P : Inport
  THS : Inport  Port=2
  Gain : Gain  Gain=1/(dev.theta(4)+conv.theta(1))
  Gain1 : Gain  Gain=1/dev.theta(3)
  Gain11 : Gain  Gain=1/dev.c(1)
  Gain2 : Gain  Gain=1/dev.c(4)
  Gain3 : Gain  Gain=1/dev.theta(3)
  Gain4 : Gain  Gain=1/dev.theta(2)
  Gain5 : Gain  Gain=1/dev.c(3)
  Gain6 : Gain  Gain=1/dev.theta(2)
  Gain7 : Gain  Gain=1/dev.theta(1)
  Gain8 : Gain  Gain=1/dev.c(2)
  Gain9 : Gain  Gain=1/dev.theta(1)
  Integrator{,1..3} (4 alike) : Integrator  InitialCondition=conv.T_init-273.15
  Subtract{,1..9,11} (11 alike) : Sum  Inputs=+-
  T_c : Outport
  T_j : Outport  Port=2
  wires:
  [T2] -> Subtract4/1, Subtract6/1, Subtract7/2, Subtract9/2  "T2"
  Gain/1 -> Subtract2/2
  Subtract5/1 -> Gain5/1
  Gain4/1 -> Subtract5/1
  Subtract3/1 -> Gain3/1
  Gain8/1 -> Integrator1/1  "d_T2"
  Integrator/1 -> T_j/1, [T1]  "T1"
  [T3] -> Subtract1/1, Subtract3/1, Subtract4/2, Subtract6/2  "T3"
  P/1 -> Subtract11/1
  Subtract9/1 -> Gain9/1
  Subtract1/1 -> Gain1/1
  [T1] -> Subtract9/1, Subtract7/1  "T1"
  Integrator1/1 -> [T2]  "T2"
  Subtract/1 -> Gain/1
  [T4] -> Subtract/1, Subtract1/2, Subtract3/2  "T4"
  Subtract7/1 -> Gain7/1
  Subtract4/1 -> Gain4/1
  Integrator3/1 -> [T4], T_c/1  "T4"
  Gain2/1 -> Integrator3/1  "d_T4"
  Subtract8/1 -> Gain8/1
  THS/1 -> Subtract/2
  Gain1/1 -> Subtract2/1
  Gain9/1 -> Subtract11/2
  Gain3/1 -> Subtract5/2
  Integrator2/1 -> [T3]  "T3"
  Gain5/1 -> Integrator2/1  "d_T3"
  Gain11/1 -> Integrator/1  "d_T1"
  Subtract2/1 -> Gain2/1
  Subtract6/1 -> Gain6/1
  Subtract11/1 -> Gain11/1
  Gain7/1 -> Subtract8/1
  Gain6/1 -> Subtract8/2

== system mpm_blocks/MOSFET w// Integrated Diode 2-Level VSC/Calculate Duty & Currents/Duty Cycle Estimation ==
  v_dc : Inport
  v_s : Inport  Port=2
  Constant : Constant
  Constant2 : Constant
  Constant3 : Constant  Value=2*conv.t_d*conv.f_sw
  Constant4 : Constant  Value=2*conv.t_d*conv.f_sw
  Divide : Product  Inputs=*/
  Gain : Gain  Gain=1/2
  Gain2 : Gain  Gain=2
  MATLAB Function : MATLAB Function  TreatAsAtomicUnit=on
  MATLAB Function3 : MATLAB Function  TreatAsAtomicUnit=on
  Mux : Mux  Inputs=[3 3]
  Subtract : Sum  Inputs=-+-
  Sum1 : Sum  Inputs=+-+
  d_M : Outport
  d_D : Outport  Port=2
  wires:
  MATLAB Function3/1(y) -> Sum1/3
  Constant/1 -> Sum1/1
  v_s/1 -> Gain2/1  "v_s"
  Constant2/1 -> Subtract/2
  Gain/1 -> Subtract/1, Mux/1, MATLAB Function/1(d1)  "d_H"
  Divide/1 -> MATLAB Function3/1(u)  "m_a"
  Sum1/1 -> Gain/1
  Constant4/1 -> MATLAB Function/3(d3), d_D/1, Subtract/3  "d_D"
  Subtract/1 -> Mux/2, MATLAB Function/2(d2)  "d_L"
  Constant3/1 -> Sum1/2
  Mux/1 -> d_M/1
  Gain2/1 -> Divide/1
  v_dc/1 -> Divide/2

== system mpm_blocks/MOSFET w// Integrated Diode 2-Level VSC/Thermal Model/Subsystem1 ==
  P : Inport
  THS : Inport  Port=2
  Gain : Gain  Gain=1/(conv.dev(1).theta(4)+conv.theta(1))
  Gain1 : Gain  Gain=1/conv.dev(1).theta(3)
  Gain11 : Gain  Gain=1/conv.dev(1).c(1)
  Gain2 : Gain  Gain=1/conv.dev(1).c(4)
  Gain3 : Gain  Gain=1/conv.dev(1).theta(3)
  Gain4 : Gain  Gain=1/conv.dev(1).theta(2)
  Gain5 : Gain  Gain=1/conv.dev(1).c(3)
  Gain6 : Gain  Gain=1/conv.dev(1).theta(2)
  Gain7 : Gain  Gain=1/conv.dev(1).theta(1)
  Gain8 : Gain  Gain=1/conv.dev(1).c(2)
  Gain9 : Gain  Gain=1/conv.dev(1).theta(1)
  Integrator{,1..3} (4 alike) : Integrator  InitialCondition=conv.T_init-273.15
  Subtract{,1..9,11} (11 alike) : Sum  Inputs=+-
  T_c : Outport
  T_j : Outport  Port=2
  wires:
  [T2] -> Subtract4/1, Subtract6/1, Subtract7/2, Subtract9/2  "T2"
  Gain/1 -> Subtract2/2
  Subtract5/1 -> Gain5/1
  Gain4/1 -> Subtract5/1
  Subtract3/1 -> Gain3/1
  Gain8/1 -> Integrator1/1  "d_T2"
  Integrator/1 -> T_j/1, [T1]  "T1"
  [T3] -> Subtract1/1, Subtract3/1, Subtract4/2, Subtract6/2  "T3"
  P/1 -> Subtract11/1
  Subtract9/1 -> Gain9/1
  Subtract1/1 -> Gain1/1
  [T1] -> Subtract9/1, Subtract7/1  "T1"
  Integrator1/1 -> [T2]  "T2"
  Subtract/1 -> Gain/1
  [T4] -> Subtract/1, Subtract1/2, Subtract3/2  "T4"
  Subtract7/1 -> Gain7/1
  Subtract4/1 -> Gain4/1
  Integrator3/1 -> [T4], T_c/1  "T4"
  Gain2/1 -> Integrator3/1  "d_T4"
  Subtract8/1 -> Gain8/1
  THS/1 -> Subtract/2
  Gain1/1 -> Subtract2/1
  Gain9/1 -> Subtract11/2
  Gain3/1 -> Subtract5/2
  Integrator2/1 -> [T3]  "T3"
  Gain5/1 -> Integrator2/1  "d_T3"
  Gain11/1 -> Integrator/1  "d_T1"
  Subtract2/1 -> Gain2/1
  Subtract6/1 -> Gain6/1
  Subtract11/1 -> Gain11/1
  Gain7/1 -> Subtract8/1
  Gain6/1 -> Subtract8/2

== system mpm_blocks/MOSFET w// Integrated Diode 2-Level VSC/Thermal Model/Subsystem2 ==
  P : Inport
  THS : Inport  Port=2
  Gain : Gain  Gain=1/(conv.dev(1).theta(4)+conv.theta(1))
  Gain1 : Gain  Gain=1/conv.dev(1).theta(3)
  Gain11 : Gain  Gain=1/conv.dev(1).c(1)
  Gain2 : Gain  Gain=1/conv.dev(1).c(4)
  Gain3 : Gain  Gain=1/conv.dev(1).theta(3)
  Gain4 : Gain  Gain=1/conv.dev(1).theta(2)
  Gain5 : Gain  Gain=1/conv.dev(1).c(3)
  Gain6 : Gain  Gain=1/conv.dev(1).theta(2)
  Gain7 : Gain  Gain=1/conv.dev(1).theta(1)
  Gain8 : Gain  Gain=1/conv.dev(1).c(2)
  Gain9 : Gain  Gain=1/conv.dev(1).theta(1)
  Integrator{,1..3} (4 alike) : Integrator  InitialCondition=conv.T_init-273.15
  Subtract{,1..9,11} (11 alike) : Sum  Inputs=+-
  T_c : Outport
  T_j : Outport  Port=2
  wires:
  [T2] -> Subtract4/1, Subtract6/1, Subtract7/2, Subtract9/2  "T2"
  Gain/1 -> Subtract2/2
  Subtract5/1 -> Gain5/1
  Gain4/1 -> Subtract5/1
  Subtract3/1 -> Gain3/1
  Gain8/1 -> Integrator1/1  "d_T2"
  Integrator/1 -> T_j/1, [T1]  "T1"
  [T3] -> Subtract1/1, Subtract3/1, Subtract4/2, Subtract6/2  "T3"
  P/1 -> Subtract11/1
  Subtract9/1 -> Gain9/1
  Subtract1/1 -> Gain1/1
  [T1] -> Subtract9/1, Subtract7/1  "T1"
  Integrator1/1 -> [T2]  "T2"
  Subtract/1 -> Gain/1
  [T4] -> Subtract/1, Subtract1/2, Subtract3/2  "T4"
  Subtract7/1 -> Gain7/1
  Subtract4/1 -> Gain4/1
  Integrator3/1 -> [T4], T_c/1  "T4"
  Gain2/1 -> Integrator3/1  "d_T4"
  Subtract8/1 -> Gain8/1
  THS/1 -> Subtract/2
  Gain1/1 -> Subtract2/1
  Gain9/1 -> Subtract11/2
  Gain3/1 -> Subtract5/2
  Integrator2/1 -> [T3]  "T3"
  Gain5/1 -> Integrator2/1  "d_T3"
  Gain11/1 -> Integrator/1  "d_T1"
  Subtract2/1 -> Gain2/1
  Subtract6/1 -> Gain6/1
  Subtract11/1 -> Gain11/1
  Gain7/1 -> Subtract8/1
  Gain6/1 -> Subtract8/2

== system mpm_blocks/MOSFET w// Integrated Diode 2-Level VSC/Thermal Model/Subsystem3 ==
  P : Inport
  THS : Inport  Port=2
  Gain : Gain  Gain=1/(conv.dev(1).theta(4)+conv.theta(1))
  Gain1 : Gain  Gain=1/conv.dev(1).theta(3)
  Gain11 : Gain  Gain=1/conv.dev(1).c(1)
  Gain2 : Gain  Gain=1/conv.dev(1).c(4)
  Gain3 : Gain  Gain=1/conv.dev(1).theta(3)
  Gain4 : Gain  Gain=1/conv.dev(1).theta(2)
  Gain5 : Gain  Gain=1/conv.dev(1).c(3)
  Gain6 : Gain  Gain=1/conv.dev(1).theta(2)
  Gain7 : Gain  Gain=1/conv.dev(1).theta(1)
  Gain8 : Gain  Gain=1/conv.dev(1).c(2)
  Gain9 : Gain  Gain=1/conv.dev(1).theta(1)
  Integrator{,1..3} (4 alike) : Integrator  InitialCondition=conv.T_init-273.15
  Subtract{,1..9,11} (11 alike) : Sum  Inputs=+-
  T_c : Outport
  T_j : Outport  Port=2
  wires:
  [T2] -> Subtract4/1, Subtract6/1, Subtract7/2, Subtract9/2  "T2"
  Gain/1 -> Subtract2/2
  Subtract5/1 -> Gain5/1
  Gain4/1 -> Subtract5/1
  Subtract3/1 -> Gain3/1
  Gain8/1 -> Integrator1/1  "d_T2"
  Integrator/1 -> T_j/1, [T1]  "T1"
  [T3] -> Subtract1/1, Subtract3/1, Subtract4/2, Subtract6/2  "T3"
  P/1 -> Subtract11/1
  Subtract9/1 -> Gain9/1
  Subtract1/1 -> Gain1/1
  [T1] -> Subtract9/1, Subtract7/1  "T1"
  Integrator1/1 -> [T2]  "T2"
  Subtract/1 -> Gain/1
  [T4] -> Subtract/1, Subtract1/2, Subtract3/2  "T4"
  Subtract7/1 -> Gain7/1
  Subtract4/1 -> Gain4/1
  Integrator3/1 -> [T4], T_c/1  "T4"
  Gain2/1 -> Integrator3/1  "d_T4"
  Subtract8/1 -> Gain8/1
  THS/1 -> Subtract/2
  Gain1/1 -> Subtract2/1
  Gain9/1 -> Subtract11/2
  Gain3/1 -> Subtract5/2
  Integrator2/1 -> [T3]  "T3"
  Gain5/1 -> Integrator2/1  "d_T3"
  Gain11/1 -> Integrator/1  "d_T1"
  Subtract2/1 -> Gain2/1
  Subtract6/1 -> Gain6/1
  Subtract11/1 -> Gain11/1
  Gain7/1 -> Subtract8/1
  Gain6/1 -> Subtract8/2
